simulink model "model_1"  (R2021b)
settings: Solver=VariableStepAuto  StartTime=0.0  StopTime=5  RelTol=1e-3
values from neighbouring files (symbols this model uses):
  A = [-5, 0; 0, -10]    [task_1.m]    (also in task_3.m = [0,1;0,0]; task_4.m = [0,1;0,0]; task_5.m = [0,1;0,0]; task_6.m = [0,1;0,0])
  B = [1; 1]    [task_1.m]
  C = [1, -1; 1, 1]    [task_1.m]
settings Model: Creator=vital  LastModifiedBy=vital

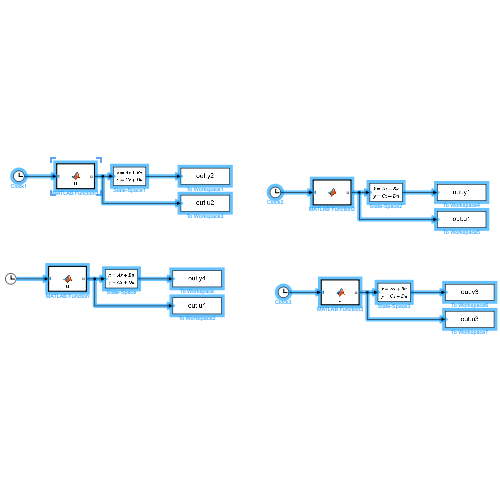
[thumbnail: Simulink's stored preview of the top-level diagram]
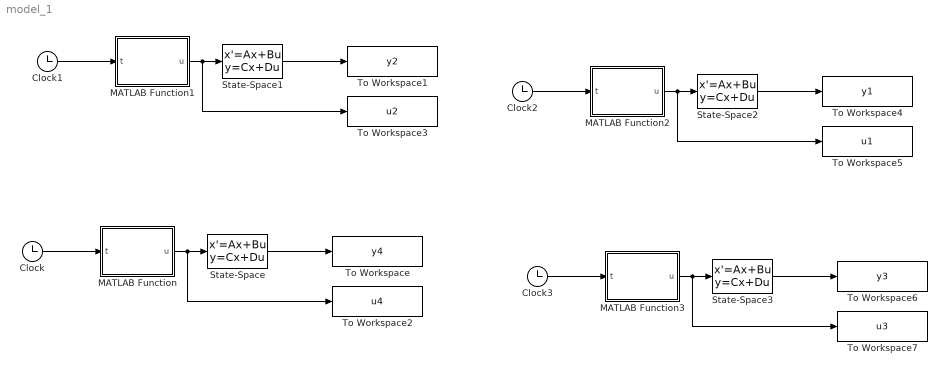
== system model_1 ==
  Clock{,1..3} (4 alike) : Clock
  MATLAB Function : MATLAB Function  TreatAsAtomicUnit=on
  MATLAB Function1 : MATLAB Function  TreatAsAtomicUnit=on
  MATLAB Function2 : MATLAB Function  TreatAsAtomicUnit=on
  MATLAB Function3 : MATLAB Function  TreatAsAtomicUnit=on
  State-Space : StateSpace  A=A  B=B  C=C  D=[0; 0]  InitialCondition=0  ParameterTunability=Optimized
  State-Space1 : StateSpace  A=A  B=B  C=C  D=[0; 0]  InitialCondition=0
  State-Space2 : StateSpace  A=A  B=B  C=C  D=[0; 0]  InitialCondition=0
  State-Space3 : StateSpace  A=A  B=B  C=C  D=[0; 0]  InitialCondition=0  ParameterTunability=Unconstrained
  To Workspace : ToWorkspace  VariableName=y4  SaveFormat=Timeseries  SampleTime=0.0005
  To Workspace1 : ToWorkspace  VariableName=y2  SaveFormat=Timeseries  SampleTime=0.0005
  To Workspace2 : ToWorkspace  VariableName=u4  SaveFormat=Timeseries  SampleTime=0.0005
  To Workspace3 : ToWorkspace  VariableName=u2  SaveFormat=Timeseries  SampleTime=0.0005
  To Workspace4 : ToWorkspace  VariableName=y1  SaveFormat=Timeseries  SampleTime=0.0005
  To Workspace5 : ToWorkspace  VariableName=u1  SaveFormat=Timeseries  SampleTime=0.0005
  To Workspace6 : ToWorkspace  VariableName=y3  SaveFormat=Timeseries  SampleTime=0.0005
  To Workspace7 : ToWorkspace  VariableName=u3  SaveFormat=Timeseries  SampleTime=0.0005
  wires:
  MATLAB Function/1(u) -> To Workspace2/1, State-Space/1
  Clock/1 -> MATLAB Function/1(t)
  State-Space/1 -> To Workspace/1
  State-Space1/1 -> To Workspace1/1
  Clock1/1 -> MATLAB Function1/1(t)
  MATLAB Function1/1(u) -> To Workspace3/1, State-Space1/1
  State-Space2/1 -> To Workspace4/1
  Clock2/1 -> MATLAB Function2/1(t)
  MATLAB Function2/1(u) -> To Workspace5/1, State-Space2/1
  State-Space3/1 -> To Workspace6/1
  Clock3/1 -> MATLAB Function3/1(t)
  MATLAB Function3/1(u) -> To Workspace7/1, State-Space3/1

== matlab function model_1/MATLAB Function ==
  data: t input; u output
function u = u(t)

if t < 0.526838
    y = (exp(5*t - 5)*(4223257209389371*exp(5*t - 5) - 2111912383887378))/70368744177664;
else
    y = 0;
end

u = y;

== matlab function model_1/MATLAB Function2 ==
  data: t input; u output
function u = u(t)

if t < 1
    y = 1;
else
    y = 0;
end

u = y;

== matlab function model_1/MATLAB Function3 ==
  data: t input; u output
function u = u(t)

y = exp(-0.5*t);

u = y;

== matlab function model_1/MATLAB Function1 ==
  data: t input; u output
function u = u(t)

if t < 0.25
    y = sqrt(8*t+3);
else
    y = 0;
end

u = y;
